simulink model "chydrbf_bruite_z"  (R2025b)
settings: Solver=ode45  StartTime=0.0  StopTime=50  MaxStep=1  MinStep=0.0001  RelTol=1e-8  AbsTol=1e-8  EnableMultiTasking=on
values from neighbouring files (symbols this model uses):
  Fd = poly(exp(Te*roots(F)))    [initchydr_yuwch.m]
  kw = 0.5    [datahydr_pprTf5.mat]    (also in initchydr_yuwch.m)
  Sd = conv(SLd,[1 -1])    [initchydr_yuwch.m]
  Ta = 10    [datahydr_pprTf5.mat]    (also in initchydr_yuwch.m)
  Td = Fd*sum(Cd)/sum(Bd)    [initchydr_yuwch.m]
  Te = 0.4    [initchydr_yuwch.m]
  TI = 0.3    [datahydr_pprTf5.mat]    (also in initchydr_yuwch.m)
  Tw = 1    [datahydr_pprTf5.mat]    (also in initchydr_yuwch.m)
undefined symbols (not defined in the file or in its folder): Rd
settings Model: Creator=pchevrel  LastModifiedBy=flo
settings SolverCC: AutoScaleAbsTol=off  AlgebraicLoopSolver=TrustRegion
settings DataIOCC: LimitDataPoints=on  SaveFormat=Array  SignalLoggingSaveFormat=ModelDataLogs  SaveOutput=off  SaveTime=off  ReturnWorkspaceOutputs=off  SignalLoggingName=sigsOut
settings OptimizationCC: ExpressionDepthLimit=2147483647.0  InitFltsAndDblsToZero=on  LifeSpan=inf
settings DebuggingCC: SaveWithParameterizedLinksMsg=none  UnderspecifiedInitializationDetection=Classic  MergeDetectMultiDrivingBlocksExec=none  SignalResolutionControl=TryResolveAllWithWarning  MultiTaskDSMMsg=warning  MultiTaskCondExecSysMsg=none  FcnCallInpInsideContextMsg=warning  UnconnectedInputMsg=warning  UnconnectedOutputMsg=warning  UnconnectedLineMsg=warning  StateNameClashWarn=warning  SFUnexpectedBacktrackingDiag=warning  SFNoUnconditionalDefaultTransitionDiag=warning  SFExecutionAtInitializationDiag=none  ArithmeticOperatorsInVariantConditions=warning
settings HardwareCC: ProdBitPerPointer=32.0  ProdBitPerSizeT=32.0  ProdBitPerPtrDiffT=32.0  ProdLargestAtomicFloat=None  ProdIntDivRoundTo=Undefined  ProdEndianess=Unspecified  ProdWordSize=32.0  ProdHWDeviceType=32-bit Generic  TargetUnknown=on
settings ModelReferenceCC: EnableRefExpFcnMdlSchedulingChecks=on  PropagateSignalLabelsOutOfModel=off
settings SFSimCC: SimUseLocalCustomCode=off  CustomCodeUndefinedFunction=UseInterfaceOnly
settings RTWCC: RTWUseLocalCustomCode=off  GPUComputeCapability=3.5  DLArmComputeVersion=19.05
settings CodeAppCC: StateflowObjectComments=on
settings GRTTargetCC: TargetFcnLib=ansi_tfl_tmw.mat  TargetLangStandard=C89/C90 (ANSI)  CombineOutputUpdateFcns=off  GRTInterface=on
settings ConfigComp: CovMetricSettings=dw  CovSaveCumulativeToWorkspaceVar=on  CovSaveSingleToWorkspaceVar=on  CovExternalEMLEnable=off

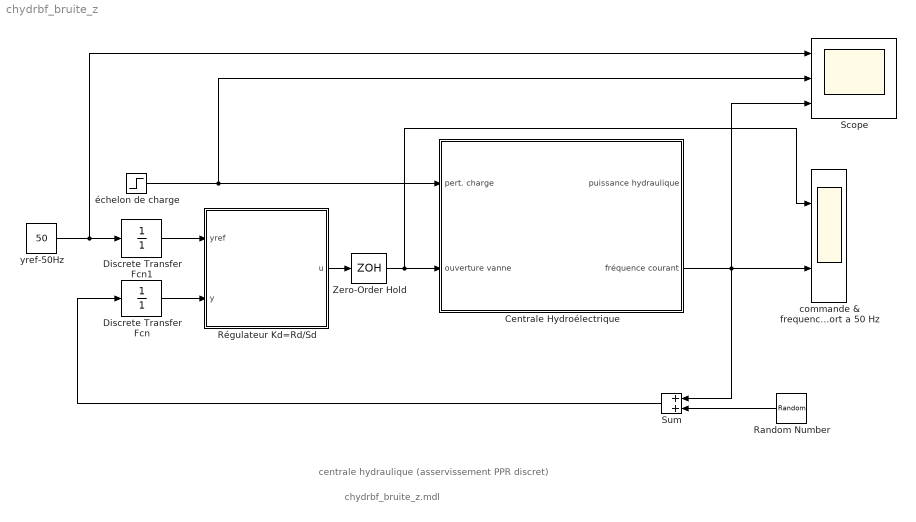
== system chydrbf_bruite_z ==
  note: chydrbf_bruite_z.mdl
  note: centrale hydraulique (asservissement PPR discret)
  Centrale Hydroélectrique : Subsystem
  Discrete Transfer Fcn : DiscreteTransferFcn  Denominator=[1]  SampleTime=Te
  Discrete Transfer Fcn1 : DiscreteTransferFcn  Denominator=[1]  SampleTime=Te
  Random Number : RandomNumber  Variance=5  SampleTime=0
  Régulateur Kd=Rd/Sd : Subsystem
  Scope : Scope  NumInputPorts=3
      settings: ActiveDisplayYMinimum=-7.0299882628759454  ActiveDisplayYMaximum=57.682578610765511
  Sum : Sum  InputSameDT=on  SaturateOnIntegerOverflow=on  OutDataTypeStr=Inherit: Same as first input
  Zero-Order Hold : ZeroOrderHold  SampleTime=Te
  commande & frequence en relatif par rapport a 50 Hz : Scope  NumInputPorts=2
      settings: ActiveDisplayYMinimum=-1  ActiveDisplayYMaximum=1
  yref-50Hz : Constant  Value=50
  échelon de charge : Step  Time=20  After=10  SampleTime=0
  wires:
  Centrale Hydroélectrique/2(fréquence courant) -> Scope/3, commande & frequence en relatif par rapport a 50 Hz/2, Sum/1
  Régulateur Kd=Rd/Sd/1(u) -> Zero-Order Hold/1
  yref-50Hz/1 -> Scope/1, Discrete Transfer Fcn1/1
  échelon de charge/1 -> Scope/2, Centrale Hydroélectrique/1(pert. charge)
  Sum/1 -> Discrete Transfer Fcn/1
  Random Number/1 -> Sum/2
  Discrete Transfer Fcn/1 -> Régulateur Kd=Rd/Sd/2(y)
  Discrete Transfer Fcn1/1 -> Régulateur Kd=Rd/Sd/1(yref)
  Zero-Order Hold/1 -> Centrale Hydroélectrique/2(ouverture vanne), commande & frequence en relatif par rapport a 50 Hz/1

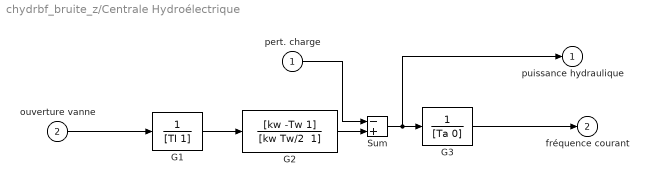
== system chydrbf_bruite_z/Centrale Hydroélectrique ==
  pert. charge : Inport
  ouverture vanne : Inport  Port=2
  G1 : TransferFcn  Denominator=[TI 1]
  G2 : TransferFcn  Numerator=[kw -Tw 1]  Denominator="[kw Tw/2  1]"
  G3 : TransferFcn  Denominator=[Ta 0]
  Sum : Sum  Inputs=-+  InputSameDT=on  SaturateOnIntegerOverflow=on  OutDataTypeStr=Inherit: Same as first input
  puissance hydraulique : Outport
  fréquence courant : Outport  Port=2
  wires:
  G2/1 -> Sum/2
  Sum/1 -> G3/1, puissance hydraulique/1
  G3/1 -> fréquence courant/1
  G1/1 -> G2/1
  pert. charge/1 -> Sum/1
  ouverture vanne/1 -> G1/1

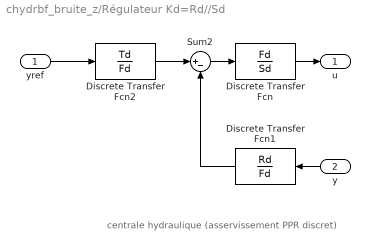
== system chydrbf_bruite_z/Régulateur Kd=Rd//Sd ==
  note: centrale hydraulique (asservissement PPR discret)
  yref : Inport
  y : Inport  Port=2
  Discrete Transfer Fcn : DiscreteTransferFcn  Numerator=Fd  Denominator=Sd  SampleTime=Te
  Discrete Transfer Fcn1 : DiscreteTransferFcn  Numerator=Rd  Denominator=Fd  SampleTime=Te
  Discrete Transfer Fcn2 : DiscreteTransferFcn  Numerator=Td  Denominator=Fd  SampleTime=Te
  Sum2 : Sum  Inputs=|+-  InputSameDT=on  SaturateOnIntegerOverflow=on  OutDataTypeStr=Inherit: Same as first input
  u : Outport
  wires:
  Sum2/1 -> Discrete Transfer Fcn/1
  Discrete Transfer Fcn2/1 -> Sum2/1
  Discrete Transfer Fcn1/1 -> Sum2/2
  yref/1 -> Discrete Transfer Fcn2/1
  Discrete Transfer Fcn/1 -> u/1
  y/1 -> Discrete Transfer Fcn1/1
